simulink library "qrd_matrix_library"  (Simulink 8.7)
settings: Solver=ode45  StartTime=0.0  StopTime=10.0  RelTol=1e-3
values from neighbouring files (symbols this model uses):
  vectorization = 2    [qrd_test.m]
undefined symbols (not defined in the file or in its folder): AdvDSPBChannelOutDisplay, AdvDSPBDMemDisplay, Back_Substitution_instances, column_count, column_count_1, column_count_2, dpoly, dspba_ChannelInVis, dspba_ChannelOutVis, dspba_internal_get_channel_ports, evalAionMaskParam, latency, primtype, QRD_vectorization, recipsqrt, row, row_count, row_count_1, row_count_2, UseDontCare, value, x
libraries: DSPBAPrim x683, DSPBAControl x37, qrd_matrix_library x33, DSPBAVectorUtil x6, DSPBAVectorPrim x3
(part 1 of 8)
settings Model: Creator=idf-2016  LastModifiedBy=5g

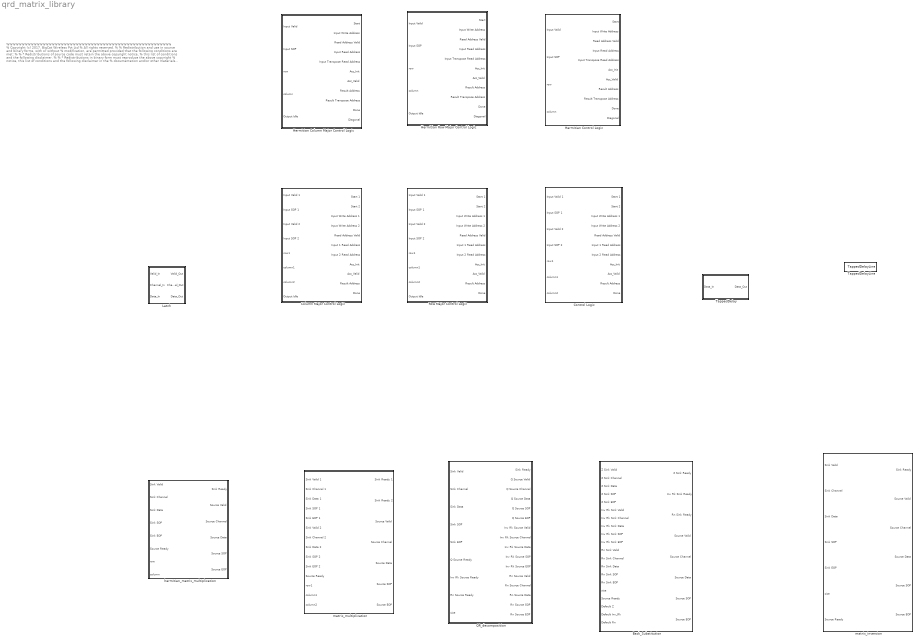
== system qrd_matrix_library ==
  note: %%%%%%%%%%%%%%%%%%%%%%%%%%%%%%%%%%%%%%%%%%%%%%%%%%%%%%%
      |  % Copyright (c) 2017, BigCat Wireless Pvt Ltd
      |  % All rights reserved.
      |  %
      |  % Redistribution and use in source and binary forms, with or without
      |  % modification, are permitted provided that the following conditions are met:
      |  %
      |  %     * Redistributions of source code must retain the above copyright notice,
      |  %       this list of conditions and the following disclaimer.
      |  %
      |  %     * Redistributions in binary form must reproduce the above copyright
      |  %       notice, this list of conditions and the following disclaimer in the
      |  %       documentation and/or other materials provided with the distribution.
      |  %
      |  %     * Neither the name of the copyright holder nor the names of its contributors
      |  %       may be used to endorse or promote products derived from this software
      |  %       without specific prior written permission.
      |  %
      |  %
      |  %
      |  % THIS SOFTWARE IS PROVIDED BY THE COPYRIGHT HOLDERS AND CONTRIBUTORS "AS IS"
      |  % AND ANY EXPRESS OR IMPLIED WARRANTIES, INCLUDING, BUT NOT LIMITED TO, THE
      |  % IMPLIED WARRANTIES OF MERCHANTABILITY AND FITNESS FOR A PARTICULAR PURPOSE ARE
      |  % DISCLAIMED. IN NO EVENT SHALL THE COPYRIGHT HOLDER OR CONTRIBUTORS BE LIABLE
      |  % FOR ANY DIRECT, INDIRECT, INCIDENTAL, SPECIAL, EXEMPLARY, OR CONSEQUENTIAL
      |  % DAMAGES (INCLUDING, BUT NOT LIMITED TO, PROCUREMENT OF SUBSTITUTE GOODS OR
      |  % SERVICES; LOSS OF USE, DATA, OR PROFITS; OR BUSINESS INTERRUPTION) HOWEVER
      |  % CAUSED AND ON ANY THEORY OF LIABILITY, WHETHER IN CONTRACT, STRICT LIABILITY,
      |  % OR TORT (INCLUDING NEGLIGENCE OR OTHERWISE) ARISING IN ANY WAY OUT OF THE USE
      |  % OF THIS SOFTWARE, EVEN IF ADVISED OF THE POSSIBILITY OF SUCH DAMAGE.
      |  %
      |   %%%%%%%%%%%%%%%%%%%%%%%%%%%%%%%%%%%%%%%%%%%%%%%%%%%%%%%%%%
  Back_Substitution : Subsystem  mask{size=16, instances=4}
      mask prompts: size "Number of Unknowns"; instances "Number of Instances"
  Column Major Control Logic : Subsystem
  Control Logic : Subsystem  BlockChoice=Row Major Control Logic
      settings: TemplateBlock=self  MemberBlocks=Column Major Control Logic,Row Major Control Logic
  Hermitian Column Major Control Logic : Subsystem
  Hermitian Control Logic : Subsystem  BlockChoice=Hermitian Column Major Control Logic
      settings: TemplateBlock=self  MemberBlocks=Hermitian Column Major Control Logic,Hermitian Row Major Control Logic
  Hermitian Row Major Control Logic : Subsystem
  Latch : Subsystem
  QR_decomposition : Subsystem  mask{size=16, vectorization=2}
      mask prompts: size "Size of Matrix"
      mask init:
      | %Output_Word_Length = get_param(gcb,'Output_Word_Length');
      | [f,e]=log2(size);
      | if(f ~= 0.5)
      |     if(vectorization~=1)
      |         vectorization = 1;
      |         set_param(gcb,'vectorization','1');
      |         uiwait(msgbox({'Vectorization not allowed for matrix size non powers of 2';'Setting vectorization to 1'},'Vectorization error','error'));
      |     end
      | end
      | 
      | if(vectorization~=1)
      |     [f,e]=log2(vectorization);
      |     if(f ~= 0.5)
      |         vectorization = 1;
      |         set_param(gcb,'vectorization','1');
      |         uiwait(msgbox({'Non power of 2 Vectorization value not allowed';'Setting vectorization to 1'},'Vectorization error','error'));
      |     elseif(vectorization > size)
      |         vectorization = column_count;
      |         set_param(gcb,'vectorization',num2str(vectorization));
      |         uiwait(msgbox({'Vectorization should be less than matrix size';'Setting vectorization equal to matrix size'},'Vectorization error','error'));
      |     end
      | end
  Row Major Control Logic : Subsystem
  TappedDelay : Subsystem  mask{numTaps=2}
      mask prompts: numTaps "Number of Taps"
      mask init:
      | block = gcb;
      | 
      | % This block modifies itself
      | set_param(block, 'MaskSelfModifiable', 'on');
      | % delete all current connections
      | delete_line(find_system(block, 'SearchDepth', 1,...
      |             'FollowLinks', 'on', 'LookUnderMasks', 'all',...
      |             'FindAll', 'on', 'Type', 'line'));
      |         
      | % If there are any SamnpleDelays, delete them
      | delay = find_system(block, 'SearchDepth', 1,...
      |             'FollowLinks', 'on', 'LookUnderMasks', 'all',...
      |             'ReferenceBlock', 'DSPBAPrim/SampleDelay');
      | if ~isempty(delay)
      |     delete_block(delay);
      | end
      | 
      | % Delete the Simulink mux (by name)
      | if ~isempty(find_system(block, 'SearchDepth', 1,...
      |             'FollowLinks', 'on', 'LookUnderMasks', 'all',...
      |             'Name', 'Mux'))
      |         delete_block([block '/Mux']);
      | end
      | 
      | % Now have an empty subsystem cleared of any previous parameterization 
      | % add in the new blocks
      | 
      | if (numTaps <= 1)
      |     % No taps
      |     add_line(block, 'Data_In/1', 'Data_Out/1', 'AUTOROUTING','ON');
      | else
      |     % First a zero-latency or single-latency latch
      |     tdspacing = min(100,(2^14)/numTaps);
      |     tdspacing_half = tdspacing/2;
      |     tdlatchheight = min(40,tdspacing);
      |     
      |     for n=1:(numTaps-1)
      |         add_block('DSPBAPrim/SampleDelay', [block '/tap' num2str(n)],'value',int2str(numTaps-n), 'Position', [130, 220 + tdspacing*n, 190, 220 + tdlatchheight + tdspacing*n]);
      |     end
      |     % Then the Simulink Mux
      |     add_block('built-in/Mux', [block '/Mux'], 'Inputs', int2str(numTaps), 'DisplayOption', 'bar');
      |     set_param([block '/Mux'], 'Position', [335, 190, 345, 190 + numTaps * tdspacing]);
      | 
      |     % Position the ports
      |     set_param([block '/Data_In'], 'Position',  [65,  135, 95,  150]);
      |     set_param([block '/Data_Out'],  'Position', [400,(180 + tdspacing_half*numTaps), 430, (195 + tdspacing_half*numTaps )]);
      | 
      | 
      |     % Now to connect - data chain
      |     add_line(block, 'Data_In/1', sprintf('Mux/%d', numTaps), 'AUTOROUTING','ON');
      |     for n=1:(numTaps-1)
      |         add_line(block, 'Data_In/1', sprintf('tap%d/1', n), 'AUTOROUTING','ON');
      |     end
      | 
      |     % Now to connect the mux to the output
      |     add_line(block, 'Mux/1', 'Data_Out/1');
      |  
      |     % Now to connect - chain to mux
      |     for n=1:(numTaps-1)
      |         add_line(block, sprintf('tap%d/1', n), sprintf('Mux/%d', n));
      |     end
      | end
  TappedDelayLine : DSPBAVectorUtil/TappedDelayLine  numTaps=Back_Substitution_instances/QRD_vectorization  zeroOrOne=0  reverse=on
  hermitian_matrix_multiplication : Subsystem  mask{row_count=16, column_count=32, vectorization=2, output_order=Row Major}
      mask prompts: row_count "Number of Rows"; column_count "Number of Columns"; output_order "Output order"
      mask init:
      | %Output_Word_Length = get_param(gcb,'Output_Word_Length');
      | [f,e]=log2(column_count);
      | if(f ~= 0.5)
      |     if(vectorization~=1)
      |         vectorization = 1;
      |         set_param(gcb,'vectorization','1');
      |         uiwait(msgbox({'Vectorization not allowed for column count non powers of 2';'Setting vectorization to 1'},'Vectorization error','error'));
      |     end
      | end
      | 
      | if(vectorization~=1)
      |     [f,e]=log2(vectorization);
      |     if(f ~= 0.5)
      |         vectorization = 1;
      |         set_param(gcb,'vectorization','1');
      |         uiwait(msgbox({'Non power of 2 Vectorization value not allowed';'Setting vectorization to 1'},'Vectorization error','error'));
      |     elseif(vectorization > column_count)
      |         vectorization = column_count;
      |         set_param(gcb,'vectorization',num2str(vectorization));
      |         uiwait(msgbox({'Vectorization should be less than column count';'Setting vectorization equal to column count'},'Vectorization error','error'));
      |     end
      | end
      | 
      | if(output_order==1)
      |     set_param([gcb '/Hermitian Control Logic'],'BlockChoice','Hermitian Row Major Control Logic');
      | elseif(output_order==2)
      |     set_param([gcb '/Hermitian Control Logic'],'BlockChoice','Hermitian Column Major Control Logic');
      | end
      mask TypeOptions output_order: Row Major | Column Major
  matrix_inversion : Subsystem  mask{size=16, QRD_vectorization=2, Back_Substitution_instances=4}
      mask prompts: size "Size of Matrix"; QRD_vectorization "Vectorization"; Back_Substitution_instances "Number of Instances"
      mask DialogControl QRDGroupVar Prompt: QR Decomposition
      mask DialogControl BSGroupVar Prompt: BackSubstitution
  matrix_multiplication : Subsystem  mask{row_count_1=16, column_count_1=16, row_count_2=16, column_count_2=32, vectorization=4, output_order=Row Major}
      mask prompts: row_count_1 "Number of Rows"; column_count_1 "Number of Columns"; row_count_2 "Number of Rows"; column_count_2 "Number of Columns"; output_order "Output order"
      mask init:
      | %Output_Word_Length = get_param(gcb,'Output_Word_Length');
      | 
      | if(column_count_1~=row_count_2)
      |     row_count_2 = column_count_1;
      |     set_param(gcb,'row_count_2',num2str(row_count_2));
      |     uiwait(msgbox({'Matrix 2 row should be equal to Matrix 1 column';'Setting Matrix 2 row equal to Matrix 1 column'},'Dimension error','error'));
      | end
      | 
      | [f,e]=log2(column_count_1);
      | if(f ~= 0.5)
      |     if(vectorization~=1)
      |         vectorization = 1;
      |         set_param(gcb,'vectorization','1');
      |         uiwait(msgbox({'Vectorization not allowed for Matrix 1 column count non powers of 2';'Setting vectorization to 1'},'Vectorization error','error'));
      |     end
      | end
      | 
      | if(vectorization~=1)
      |     [f,e]=log2(vectorization);
      |     if(f ~= 0.5)
      |         vectorization = 1;
      |         set_param(gcb,'vectorization','1');
      |         uiwait(msgbox({'Non power of 2 Vectorization value not allowed';'Setting vectorization to 1'},'Vectorization error','error'));
      |     elseif(vectorization > column_count_1)
      |         vectorization = column_count_1;
      |         set_param(gcb,'vectorization',num2str(vectorization));
      |         uiwait(msgbox({'Vectorization should be less than Matrix 1 column count';'Setting vectorization equal to column count'},'Vectorization error','error'));
      |     end
      | end
      | 
      | if(output_order==1)
      |     set_param([gcb '/Control Logic'],'BlockChoice','Row Major Control Logic');
      | elseif(output_order==2)
      |     set_param([gcb '/Control Logic'],'BlockChoice','Column Major Control Logic');
      | end
      mask TypeOptions output_order: Row Major | Column Major
      mask DialogControl Matrix1GroupVar Prompt: Matrix 1
      mask DialogControl Matrix2GroupVar Prompt: Matrix 2

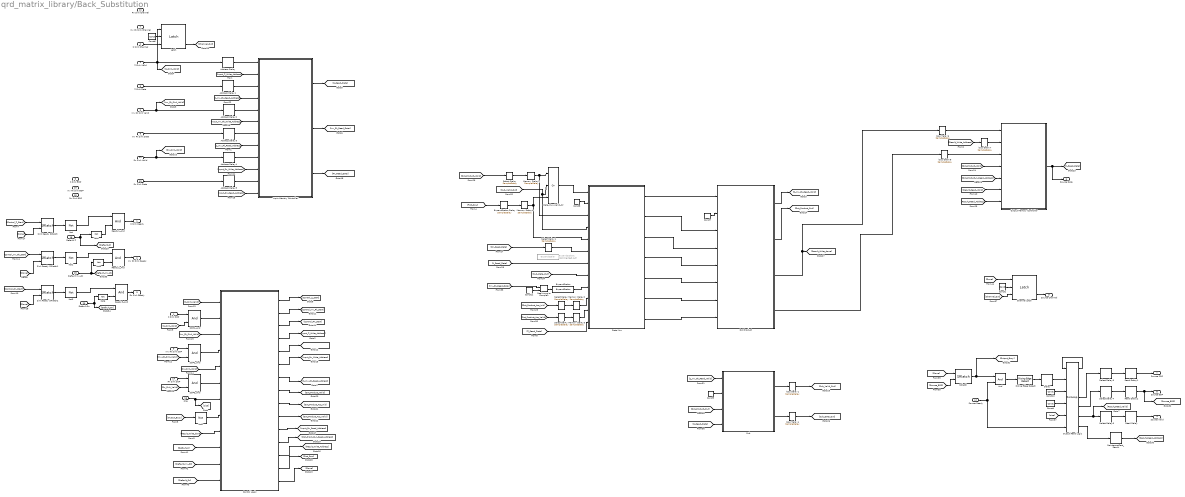
== system qrd_matrix_library/Back_Substitution ==
  Z Sink Valid : Inport
  Z Sink Channel : Inport  Port=2
  Z Sink Data : Inport  Port=3
  Z Sink SOP : Inport  Port=4
  Z Sink EOP : Inport  Port=5
  Inv Rk Sink Valid : Inport  Port=6
  Inv Rk Sink Channel : Inport  Port=7
  Inv Rk Sink Data : Inport  Port=8
  Inv Rk Sink SOP : Inport  Port=9
  Inv Rk Sink EOP : Inport  Port=10
  Rn Sink Valid : Inport  Port=11
  Rn Sink Channel : Inport  Port=12
  Rn Sink Data : Inport  Port=13
  Rn Sink SOP : Inport  Port=14
  Rn Sink EOP : Inport  Port=15
  size : Inport  Port=16
  Source Ready : Inport  Port=17
  Default Z : Inport  Port=18
  Default Inv_Rk : Inport  Port=19
  Default Rn : Inport  Port=20
  Address Delay{,1..5} (6 alike) : DSPBAPrim/SampleDelay  primtype=sampdelay  nInputs=1  nOutputs=1  omode=Inherit via internal rule  otype=sfix(16)  scale=2^-15  rndmethod=Unbiased  factor=1  satmethod=Symmetric  shift_vec=[0 1 2 -1]  value=1  inPortNames=[' '; ' ';]  outPortNames=[' ']  dspbaimage=dspba_prim.jpg  text=dpoly(1, eye(1,value+1), 'z')  style=Optimised  visibilities=8 + 1024 + 2^17 + 2^18  flexible=off  slackgroup=0  augmented=0  version=20090407  advOptions=[]
  And : DSPBAPrim/And  primtype=and  nInputs=2  nOutputs=1  omode=Inherit via internal rule  otype=sfix(16)  scale=2^-15  rndmethod=Unbiased  factor=1  satmethod=Symmetric  shift_vec=[0 1 2 -1]  value=0  inPortNames=[' '; ' '; ' '; ' '; ' '; ' '; ' '; ' '; ' '; ' '; ' '; ' '; ' '; ' '; ' '; ' '; ]  outPortNames=[' ']  dspbaimage=dspba_prim.jpg  text=fprintf('&');  style=Optimised  visibilities=8+2  version=20090407
  Channel Latch : qrd_matrix_library/Latch
  Const{1,6..9} (5 alike) : DSPBAPrim/Const  primtype=const  nInputs=0  nOutputs=1  omode=Specify via dialog  otype=uint(8)  scale=1  rndmethod=Unbiased  factor=1  satmethod=Symmetric  shift_vec=[0 1 2 -1]  value=0  inPortNames=['+'; '+';]  outPortNames=[' ']  dspbaimage=dspba_prim.jpg  text=fprintf('%s', num2str(value));  style=Optimised  visibilities=8 + 1024  floatPrecision=float32_m23  version=20120820
  Const10 : DSPBAPrim/Const  primtype=const  nInputs=0  nOutputs=1  omode=Specify via dialog  otype=uint(nextpow2(size))  scale=1  rndmethod=Unbiased  factor=1  satmethod=Symmetric  shift_vec=[0 1 2 -1]  value=0  inPortNames=['+'; '+';]  outPortNames=[' ']  dspbaimage=dspba_prim.jpg  text=fprintf('%s', num2str(value));  style=Optimised  visibilities=8 + 1024  floatPrecision=float32_m23  version=20120820
  Const11 : DSPBAPrim/Const  primtype=const  nInputs=0  nOutputs=1  omode=single  otype=uint(8)  scale=1  rndmethod=Unbiased  factor=1  satmethod=Symmetric  shift_vec=[0 1 2 -1]  value=0  inPortNames=['+'; '+';]  outPortNames=[' ']  dspbaimage=dspba_prim.jpg  text=fprintf('%s', num2str(value));  style=Optimised  visibilities=8 + 1024  floatPrecision=float32_m23  version=20120820
  Const4 : DSPBAPrim/Const  primtype=const  nInputs=0  nOutputs=1  omode=Inherit via internal rule  otype=uint(nextpow2(row*row))  scale=1  rndmethod=Unbiased  factor=1  satmethod=Symmetric  shift_vec=[0 1 2 -1]  value=1  inPortNames=['+'; '+';]  outPortNames=[' ']  dspbaimage=dspba_prim.jpg  text=fprintf('%s', num2str(value));  style=Optimised  visibilities=8 + 1024  floatPrecision=float32_m23  version=20120820
  Control Logic : Subsystem
  Data Mux : Subsystem
  Data_Mux_Valid_Or : DSPBAPrim/Or  primtype=or  nInputs=3  nOutputs=1  omode=Inherit via internal rule  otype=sfix(16)  scale=2^-15  rndmethod=Unbiased  factor=1  satmethod=Symmetric  shift_vec=[0 1 2 -1]  value=0  inPortNames=[' '; ' '; ' '; ' '; ' '; ' '; ' '; ' '; ' '; ' '; ' '; ' '; ' '; ' '; ' '; ' '; ]  outPortNames=[' ']  dspbaimage=dspba_prim.jpg  text=fprintf('|');  style=Optimised  visibilities=8+2  version=20090407
  Delay : DSPBAPrim/SampleDelay  primtype=sampdelay  nInputs=1  nOutputs=1  omode=Inherit via internal rule  otype=sfix(16)  scale=2^-15  rndmethod=Unbiased  factor=1  satmethod=Symmetric  shift_vec=[0 1 2 -1]  value=1  inPortNames=[' '; ' ';]  outPortNames=[' ']  dspbaimage=dspba_prim.jpg  text=dpoly(1, eye(1,value+1), 'z')  style=Optimised  visibilities=8 + 1024 + 2^17 + 2^18  flexible=off  slackgroup=0  augmented=0  version=20090407  advOptions=[]
  Dot Product : Subsystem
  ExpandScalar : DSPBAVectorUtil/ExpandScalar  vecWidth=instances
  ExpandScalar Delay : DSPBAPrim/SampleDelay  primtype=sampdelay  nInputs=1  nOutputs=1  omode=Inherit via internal rule  otype=sfix(16)  scale=2^-15  rndmethod=Unbiased  factor=1  satmethod=Symmetric  shift_vec=[0 1 2 -1]  value=1  inPortNames=[' '; ' ';]  outPortNames=[' ']  dspbaimage=dspba_prim.jpg  text=dpoly(1, eye(1,value+1), 'z')  style=Optimised  visibilities=8 + 1024 + 2^17 + 2^18  flexible=off  slackgroup=0  augmented=0  version=20090407  advOptions=[]
  ExpandScalar1 : DSPBAVectorUtil/ExpandScalar  Commented=on  vecWidth=instances
  Input Memory Controller : Subsystem
  Latch : qrd_matrix_library/Latch
  Memory Delay{1..4} (4 alike) : DSPBAPrim/SampleDelay  primtype=sampdelay  nInputs=1  nOutputs=1  omode=Inherit via internal rule  otype=sfix(16)  scale=2^-15  rndmethod=Unbiased  factor=1  satmethod=Symmetric  shift_vec=[0 1 2 -1]  value=2  inPortNames=[' '; ' ';]  outPortNames=[' ']  dspbaimage=dspba_prim.jpg  text=dpoly(1, eye(1,value+1), 'z')  style=Optimised  visibilities=8 + 1024 + 2^17 + 2^18  flexible=off  slackgroup=0  augmented=0  version=20090407  advOptions=[]
  Not{,1..6} (7 alike) : DSPBAPrim/Not  primtype=not  nInputs=1  nOutputs=1  omode=Inherit via internal rule  otype=sfix(16)  scale=2^-15  rndmethod=Unbiased  factor=1  satmethod=Symmetric  shift_vec=[0 1 2 -1]  value=0  inPortNames=[' '; ' ';]  outPortNames=[' ']  dspbaimage=dspba_prim.jpg  text=fprintf('~');  style=Optimised  visibilities=8  version=20090407
  Output Memory Controller : Subsystem
  Output Read Logic : DSPBAPrim/ForLoop  looptest=<
  Read Delay : DSPBAPrim/SampleDelay  primtype=sampdelay  nInputs=1  nOutputs=1  omode=Inherit via internal rule  otype=sfix(16)  scale=2^-15  rndmethod=Unbiased  factor=1  satmethod=Symmetric  shift_vec=[0 1 2 -1]  value=2  inPortNames=[' '; ' ';]  outPortNames=[' ']  dspbaimage=dspba_prim.jpg  text=dpoly(1, eye(1,value+1), 'z')  style=Optimised  visibilities=8 + 1024 + 2^17 + 2^18  flexible=off  slackgroup=0  augmented=0  version=20090407  advOptions=[]
  Read Delay1 : DSPBAPrim/SampleDelay  primtype=sampdelay  nInputs=1  nOutputs=1  omode=Inherit via internal rule  otype=sfix(16)  scale=2^-15  rndmethod=Unbiased  factor=1  satmethod=Symmetric  shift_vec=[0 1 2 -1]  value=2  inPortNames=[' '; ' ';]  outPortNames=[' ']  dspbaimage=dspba_prim.jpg  text=dpoly(1, eye(1,value+1), 'z')  style=Optimised  visibilities=8 + 1024 + 2^17 + 2^18  flexible=off  slackgroup=0  augmented=0  version=20090407  advOptions=[]
  Read Delay2 : DSPBAPrim/SampleDelay  primtype=sampdelay  nInputs=1  nOutputs=1  omode=Inherit via internal rule  otype=sfix(16)  scale=2^-15  rndmethod=Unbiased  factor=1  satmethod=Symmetric  shift_vec=[0 1 2 -1]  value=2  inPortNames=[' '; ' ';]  outPortNames=[' ']  dspbaimage=dspba_prim.jpg  text=dpoly(1, eye(1,value+1), 'z')  style=Optimised  visibilities=8 + 1024 + 2^17 + 2^18  flexible=off  slackgroup=0  augmented=0  version=20090407  advOptions=[]
  Ready1_And : DSPBAPrim/And  primtype=and  nInputs=2  nOutputs=1  omode=Inherit via internal rule  otype=sfix(16)  scale=2^-15  rndmethod=Unbiased  factor=1  satmethod=Symmetric  shift_vec=[0 1 2 -1]  value=0  inPortNames=[' '; ' '; ' '; ' '; ' '; ' '; ' '; ' '; ' '; ' '; ' '; ' '; ' '; ' '; ' '; ' '; ]  outPortNames=[' ']  dspbaimage=dspba_prim.jpg  text=fprintf('&');  style=Optimised  visibilities=8+2  version=20090407
  Ready2_And : DSPBAPrim/And  primtype=and  nInputs=2  nOutputs=1  omode=Inherit via internal rule  otype=sfix(16)  scale=2^-15  rndmethod=Unbiased  factor=1  satmethod=Symmetric  shift_vec=[0 1 2 -1]  value=0  inPortNames=[' '; ' '; ' '; ' '; ' '; ' '; ' '; ' '; ' '; ' '; ' '; ' '; ' '; ' '; ' '; ' '; ]  outPortNames=[' ']  dspbaimage=dspba_prim.jpg  text=fprintf('&');  style=Optimised  visibilities=8+2  version=20090407
  Ready3_And : DSPBAPrim/And  primtype=and  nInputs=2  nOutputs=1  omode=Inherit via internal rule  otype=sfix(16)  scale=2^-15  rndmethod=Unbiased  factor=1  satmethod=Symmetric  shift_vec=[0 1 2 -1]  value=0  inPortNames=[' '; ' '; ' '; ' '; ' '; ' '; ' '; ' '; ' '; ' '; ' '; ' '; ' '; ' '; ' '; ' '; ]  outPortNames=[' ']  dspbaimage=dspba_prim.jpg  text=fprintf('&');  style=Optimised  visibilities=8+2  version=20090407
  Real-Imag to Complex : RealImagToComplex
  ReinterpretCast_Result : DSPBAPrim/ReinterpretCast  primtype=reinterpret  nInputs=1  nOutputs=1  omode=Specify via dialog  otype=uint(nextpow2(size))  scale=1  rndmethod=Unbiased  factor=1  satmethod=Symmetric  shift_vec=[0 1 2 -1]  value=0  inPortNames=[' '; ' ';]  outPortNames=[' ']  dspbaimage=dspba_prim.jpg  text=fprintf('Reinterp\nCast', value);  style=Optimised  visibilities=8  floatPrecision=float32_m23  version=20120601
  Rising Edge Detect : qrd_matrix_library/matrix_multiplication/Rising Edge Detect
  SOP1_And : DSPBAPrim/And  primtype=and  nInputs=2  nOutputs=1  omode=Inherit via internal rule  otype=sfix(16)  scale=2^-15  rndmethod=Unbiased  factor=1  satmethod=Symmetric  shift_vec=[0 1 2 -1]  value=0  inPortNames=[' '; ' '; ' '; ' '; ' '; ' '; ' '; ' '; ' '; ' '; ' '; ' '; ' '; ' '; ' '; ' '; ]  outPortNames=[' ']  dspbaimage=dspba_prim.jpg  text=fprintf('&');  style=Optimised  visibilities=8+2  version=20090407
  SOP2_And : DSPBAPrim/And  primtype=and  nInputs=2  nOutputs=1  omode=Inherit via internal rule  otype=sfix(16)  scale=2^-15  rndmethod=Unbiased  factor=1  satmethod=Symmetric  shift_vec=[0 1 2 -1]  value=0  inPortNames=[' '; ' '; ' '; ' '; ' '; ' '; ' '; ' '; ' '; ' '; ' '; ' '; ' '; ' '; ' '; ' '; ]  outPortNames=[' ']  dspbaimage=dspba_prim.jpg  text=fprintf('&');  style=Optimised  visibilities=8+2  version=20090407
  SOP3_And : DSPBAPrim/And  primtype=and  nInputs=2  nOutputs=1  omode=Inherit via internal rule  otype=sfix(16)  scale=2^-15  rndmethod=Unbiased  factor=1  satmethod=Symmetric  shift_vec=[0 1 2 -1]  value=0  inPortNames=[' '; ' '; ' '; ' '; ' '; ' '; ' '; ' '; ' '; ' '; ' '; ' '; ' '; ' '; ' '; ' '; ]  outPortNames=[' ']  dspbaimage=dspba_prim.jpg  text=fprintf('&');  style=Optimised  visibilities=8+2  version=20090407
  SRlatch : DSPBAControl/SRlatch
  Select Delay{,1..6} (7 alike) : DSPBAPrim/SampleDelay  primtype=sampdelay  nInputs=1  nOutputs=1  omode=Inherit via internal rule  otype=sfix(16)  scale=2^-15  rndmethod=Unbiased  factor=1  satmethod=Symmetric  shift_vec=[0 1 2 -1]  value=1  inPortNames=[' '; ' ';]  outPortNames=[' ']  dspbaimage=dspba_prim.jpg  text=dpoly(1, eye(1,value+1), 'z')  style=Optimised  visibilities=8 + 1024 + 2^17 + 2^18  flexible=off  slackgroup=0  augmented=0  version=20090407  advOptions=[]
  Sink Ready SRlatch : DSPBAControl/SRlatch
  Sink Ready SRlatch1 : DSPBAControl/SRlatch
  Sink Ready SRlatch2 : DSPBAControl/SRlatch
  Sub : Subsystem
  loop Delay{1,4,6..8} (5 alike) : DSPBAPrim/SampleDelay  primtype=sampdelay  nInputs=1  nOutputs=1  omode=Inherit via internal rule  otype=sfix(16)  scale=2^-15  rndmethod=Unbiased  factor=1  satmethod=Symmetric  shift_vec=[0 1 2 -1]  value=1  inPortNames=[' '; ' ';]  outPortNames=[' ']  dspbaimage=dspba_prim.jpg  text=dpoly(1, eye(1,value+1), 'z')  style=Optimised  visibilities=8 + 1024 + 2^17 + 2^18  flexible=off  slackgroup=0  augmented=0  version=20090407  advOptions=[]
  Z Sink Ready : Outport
  Inv Rk Sink Ready : Outport  Port=2
  Rn Sink Ready : Outport  Port=3
  Source Valid : Outport  Port=4
  Source Channel : Outport  Port=5
  Source Data : Outport  Port=6
  Source SOP : Outport  Port=7
  Source EOP : Outport  Port=8
  wires:
  Address Delay/1 -> Input Memory Controller/1(Z External Write)
  Z Sink Data/1 -> Address Delay1/1
  Control Logic/4(Z Input Write Address) -> [Input_Z_Write_Address]
  Address Delay1/1 -> Input Memory Controller/3(Z External Write Data)
  [Input_Z_Write_Address] -> Input Memory Controller/2(Z External Write Address)
  Z Sink SOP/1 -> SOP1_And/1
  [Z_Inv_Rk_Read_Address] -> Input Memory Controller/4(Z Read Address)
  [Z_Inv_Rk_Read_Address] -> Input Memory Controller/8(Inv Rk Read Address)
  Z Sink Valid/1 -> Latch/1, Address Delay/1, [Z_Sink_Valid]
  Not/1 -> Ready1_And/1
  [Done] -> Sink Ready SRlatch/2
  Z Sink Channel/1 -> Latch/3
  Const6/1 -> Latch/2
  Latch/3 -> [Channel_Out]
  Sink Ready SRlatch/1 -> Not/1
  [Z_Sink_Valid] -> SOP1_And/2
  SOP1_And/1 -> Control Logic/2(Z Input SOP)
  Control Logic/1(Z Start) -> [Control_Z_Start]
  Not1/1 -> Ready2_And/1
  [Done] -> Sink Ready SRlatch1/2
  Sink Ready SRlatch1/1 -> Not1/1
  [Control_Inv_Rk_Start] -> Sink Ready SRlatch1/1
  Address Delay2/1 -> Input Memory Controller/5(Inv Rk External Write)
  Inv Rk Sink Valid/1 -> [Inv_Rk_Sink_Valid], Address Delay2/1
  Address Delay3/1 -> Input Memory Controller/7(Inv Rk External Write Data)
  Inv Rk Sink Data/1 -> Address Delay3/1
  [Inv_Rk_Sink_Valid] -> SOP2_And/2
  Inv Rk Sink SOP/1 -> SOP2_And/1
  [Z_Sink_Valid] -> Control Logic/1(Z Input Valid)
  [Inv_Rk_Sink_Valid] -> Control Logic/3(Inv Rk Input Valid)
  SOP2_And/1 -> Control Logic/4(Inv Rk Input SOP)
  size/1 -> [size], Control Logic/7(size)
  Control Logic/2(Inv Rk Start) -> [Control_Inv_Rk_Start]
  [Input_Inv_Rk_Write_Address] -> Input Memory Controller/6(Inv Rk External Write Address)
  Control Logic/5(Inv Rk Input Write Address) -> [Input_Inv_Rk_Write_Address]
  [Output_Busy] -> Not2/1
  Not2/1 -> Control Logic/8(Output Idle)
  Rn Sink Valid/1 -> [Rn_Sink_Valid], Address Delay4/1
  Rn Sink Data/1 -> Address Delay5/1
  Address Delay4/1 -> Input Memory Controller/9(Rn External Write)
  Address Delay5/1 -> Input Memory Controller/11(Rn External Write Data)
  Not3/1 -> Ready3_And/1
  [Done] -> Sink Ready SRlatch2/2
  Sink Ready SRlatch2/1 -> Not3/1
  [Control_Rn_Start] -> Sink Ready SRlatch2/1
  [Rn_Sink_Valid] -> SOP3_And/2
  SOP3_And/1 -> Control Logic/6(Rn Input SOP)
  Rn Sink SOP/1 -> SOP3_And/1
  [Rn_Sink_Valid] -> Control Logic/5(Rn Input Valid)
  Control Logic/3(Rn Start) -> [Control_Rn_Start]
  Control Logic/6(Rn Input Write Address) -> [Input_Rn_Write_Address]
  [Input_Rn_Write_Address] -> Input Memory Controller/10(Rn External Write Address)
  Control Logic/7(Z Inv_Rk Read Address) -> [Z_Inv_Rk_Read_Address]
  [Input_Rn_Read_Address] -> Input Memory Controller/12(Rn Read Address)
  Control Logic/13(Result Write Address) -> [Result_Write_Address]
  Input Memory Controller/1(Z Data) -> [Z_Read_Data]
  Input Memory Controller/2(Inv Rk Data) -> [Inv_Rk_Read_Data]
  Control Logic/15(Done) -> [Done]
  Const7/1 -> Dot Product/2(Channel_In)
  Data Mux/4(Acc_Init_Out) -> Dot Product/5(Acc_Init)
  Data Mux/2(Data Out 1) -> Dot Product/3(Data_In1)
  Data Mux/1(Valid Out) -> Dot Product/1(Valid_In)
  Data Mux/3(Data Out 2) -> Dot Product/4(Data_In2)
  Data Mux/5(Acc_Valid_Out) -> Dot Product/6(Acc_Valid)
  Control Logic/11(Rn Read Address) -> [Input_Rn_Read_Address]
  Input Memory Controller/3(Rn Data) -> [Rn_Read_Data]
  Control Logic/12(X Read Address) -> [Dot_Product_X_Read_Address]
  Control Logic/8(Dot Product Valid) -> [Dot_Product_Valid]
  Control Logic/9(Acc_Init) -> [Dot_Product_Acc_Init]
  Control Logic/10(Acc_Valid) -> [Dot_Product_Acc_Valid]
  [Dot_Product_Valid] -> Output Memory Controller/4(Read Valid 1)
  [Result_Read_Valid] -> Output Memory Controller/6(Read Valid 2)
  [Result_Read_Address] -> Output Memory Controller/7(Read Address 2)
  [Dot_Product_X_Read_Address] -> Output Memory Controller/5(Read Address 1)
  Output Memory Controller/1(Read Data) -> Source Data/1, [X_Read_Data]
  Memory Delay1/1 -> Data Mux/3(Dot_Product_valid_in), Data_Mux_Valid_Or/1
  [Sub_Valid_Out] -> Data Mux/4(Divide_valid_in), Data_Mux_Valid_Or/2
  Data_Mux_Valid_Or/1 -> Data Mux/1(Valid In)
  Select Delay/1 -> Memory Delay1/1
  Const8/1 -> Data Mux/2(Channel In)
  Select Delay2/1 -> Memory Delay2/1
  Select Delay3/1 -> Memory Delay3/1
  Memory Delay2/1 -> Data Mux/10(Acc_Init_In)
  Memory Delay3/1 -> Data Mux/11(Acc_Valid_In)
  Dot Product/1(Dot Product Valid_Out) -> [Z_Inv_Rk_Read_Valid]
  Dot Product/2(Dot Product Data_Out) -> [Dot_Product_Out]
  [Sub_Data_Out] -> Data Mux/8(Sub_Data)
  [Inv_Rk_Read_Data] -> Real-Imag to Complex/1
  [Z_Inv_Rk_Read_Valid] -> Sub/1(Valid In)
  Const9/1 -> Sub/2(Channel In)
  [Z_Read_Data] -> Sub/4(Z_Data_In)
  [Dot_Product_Out] -> Sub/3(Acc_Data_In)
  Sub/1(Valid_out) -> loop Delay1/1
  Sub/2(Z_Acc_Data_Out) -> loop Delay4/1
  [Result_Write_done] -> Control Logic/9(Result write done)
  Data Mux/7(Divide_Valid_Out) -> Dot Product/8(Mult_Valid_In)
  Const11/1 -> Real-Imag to Complex/2
  Real-Imag to Complex/1 -> ExpandScalar/1
  ExpandScalar/1 -> Data Mux/9(Inv_Rk_Data)
  [Rn_Read_Data] -> Select Delay1/1
  Dot Product/3(Mult Valid_out) -> loop Delay6/1, [Result_Write_done]
  [Result_Write_Address] -> loop Delay7/1
  Dot Product/4(Mult Data_out) -> loop Delay8/1
  [X_Read_Data] -> Data Mux/7(X_Data)
  Select Delay1/1 -> Data Mux/6(Rn_Data)
  [Dot_Product_Valid] -> Select Delay/1
  [Dot_Product_Acc_Init] -> Select Delay2/1
  [Dot_Product_Acc_Valid] -> Select Delay3/1
  loop Delay6/1 -> Output Memory Controller/1(Write Enable)
  loop Delay7/1 -> Output Memory Controller/2(Write Address)
  loop Delay8/1 -> Output Memory Controller/3(Write Data)
  loop Delay1/1 -> [Sub_Valid_Out]
  loop Delay4/1 -> [Sub_Data_Out]
  Control Logic/14(First Row) -> [First_Row]
  Memory Delay4/1 -> Data Mux/5(First_Column_in), Data_Mux_Valid_Or/3
  ExpandScalar Delay/1 -> Memory Delay4/1
  [First_Row] -> ExpandScalar Delay/1
  [Z_Read_Data] -> Data Mux/12(Z_Data_In)
  Data Mux/6(Dot_Product_valid_out) -> Dot Product/7(Dot_Product_Valid_In)
  Read Delay1/1 -> Source SOP/1
  Read Delay/1 -> Source Valid/1
  Source Ready/1 -> Output Read Logic/6, And/2
  Read Delay2/1 -> Source EOP/1, [Source_EOP]
  Rising Edge Detect/1 -> Delay/1
  SRlatch/1 -> [Output_Busy], And/1
  And/1 -> Rising Edge Detect/1
  Delay/1 -> Output Read Logic/2
  Output Read Logic/6 -> Select Delay6/1, [Result_Read_Valid]
  Output Read Logic/7 -> ReinterpretCast_Result/1
  Output Read Logic/4 -> Select Delay5/1
  Output Read Logic/5 -> Select Delay4/1
  [size] -> Output Read Logic/5
  Const4/1 -> Output Read Logic/4
  Output Read Logic/1 -> Output Read Logic/1
  [Source_EOP] -> SRlatch/2
  ReinterpretCast_Result/1 -> [Result_Read_Address]
  [Done] -> SRlatch/1
  Select Delay5/1 -> Read Delay1/1
  Select Delay4/1 -> Read Delay2/1
  Select Delay6/1 -> Read Delay/1
  Const10/1 -> Output Read Logic/3
  Default Z/1 -> [Default_Z], Not4/1
  Default Inv_Rk/1 -> Not5/1, [Default_Inv_Rk]
  Default Rn/1 -> [Default_Rn], Not6/1
  [Default_Z] -> Control Logic/10(Default Z)
  [Default_Inv_Rk] -> Control Logic/11(Default Inv_Rk)
  [Default_Rn] -> Control Logic/12(Default Rn)
  [Control_Z_Start] -> Sink Ready SRlatch/1
  Ready1_And/1 -> Z Sink Ready/1
  Not4/1 -> Ready1_And/2
  Ready2_And/1 -> Inv Rk Sink Ready/1
  Not5/1 -> Ready2_And/2
  Ready3_And/1 -> Rn Sink Ready/1
  Not6/1 -> Ready3_And/2
  [Channel_Out] -> Channel Latch/3
  Const1/1 -> Channel Latch/2
  [Done] -> Channel Latch/1
  Channel Latch/3 -> Source Channel/1

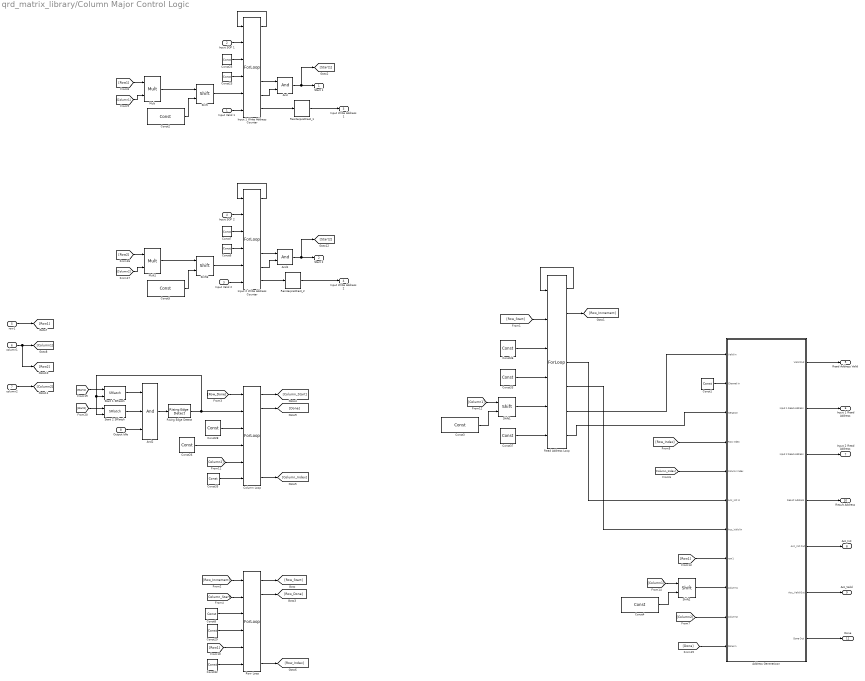
== system qrd_matrix_library/Column Major Control Logic ==
  Input Valid 1 : Inport
  Input SOP 1 : Inport  Port=2
  Input Valid 2 : Inport  Port=3
  Input SOP 2 : Inport  Port=4
  row1 : Inport  Port=5
  column1 : Inport  Port=6
  column2 : Inport  Port=7
  Output Idle : Inport  Port=8
  Address Generatioon : Subsystem
  And : DSPBAPrim/And  primtype=and  nInputs=2  nOutputs=1  omode=Inherit via internal rule  otype=sfix(16)  scale=2^-15  rndmethod=Unbiased  factor=1  satmethod=Symmetric  shift_vec=[0 1 2 -1]  value=0  inPortNames=[' '; ' '; ' '; ' '; ' '; ' '; ' '; ' '; ' '; ' '; ' '; ' '; ' '; ' '; ' '; ' '; ]  outPortNames=[' ']  dspbaimage=dspba_prim.jpg  text=fprintf('&');  style=Optimised  visibilities=8+2  version=20090407
  And1 : DSPBAPrim/And  primtype=and  nInputs=2  nOutputs=1  omode=Inherit via internal rule  otype=sfix(16)  scale=2^-15  rndmethod=Unbiased  factor=1  satmethod=Symmetric  shift_vec=[0 1 2 -1]  value=0  inPortNames=[' '; ' '; ' '; ' '; ' '; ' '; ' '; ' '; ' '; ' '; ' '; ' '; ' '; ' '; ' '; ' '; ]  outPortNames=[' ']  dspbaimage=dspba_prim.jpg  text=fprintf('&');  style=Optimised  visibilities=8+2  version=20090407
  And2 : DSPBAPrim/And  primtype=and  nInputs=3  nOutputs=1  omode=Inherit via internal rule  otype=sfix(16)  scale=2^-15  rndmethod=Unbiased  factor=1  satmethod=Symmetric  shift_vec=[0 1 2 -1]  value=0  inPortNames=[' '; ' '; ' '; ' '; ' '; ' '; ' '; ' '; ' '; ' '; ' '; ' '; ' '; ' '; ' '; ' '; ]  outPortNames=[' ']  dspbaimage=dspba_prim.jpg  text=fprintf('&');  style=Optimised  visibilities=8+2  version=20090407
  Column Loop : DSPBAPrim/ForLoop  looptest=<
  Const1 : DSPBAPrim/Const  primtype=const  nInputs=0  nOutputs=1  omode=Specify via dialog  otype=uint(8)  scale=1  rndmethod=Unbiased  factor=1  satmethod=Symmetric  shift_vec=[0 1 2 -1]  value=0  inPortNames=['+'; '+';]  outPortNames=[' ']  dspbaimage=dspba_prim.jpg  text=fprintf('%s', num2str(value));  style=Optimised  visibilities=8 + 1024  floatPrecision=float32_m23  version=20120820
  Const{2..5} (4 alike) : DSPBAPrim/Const  primtype=const  nInputs=0  nOutputs=1  omode=Inherit via internal rule  otype=uint(8)  scale=1  rndmethod=Unbiased  factor=1  satmethod=Symmetric  shift_vec=[0 1 2 -1]  value=nextpow2(vectorization)  inPortNames=['+'; '+';]  outPortNames=[' ']  dspbaimage=dspba_prim.jpg  text=fprintf('%s', num2str(value));  style=Optimised  visibilities=8 + 1024  floatPrecision=float32_m23  version=20120820
  Const{6,23,26,29,33,35,37} (7 alike) : DSPBAPrim/Const  primtype=const  nInputs=0  nOutputs=1  omode=Inherit via internal rule  otype=uint(8)  scale=1  rndmethod=Unbiased  factor=1  satmethod=Symmetric  shift_vec=[0 1 2 -1]  value=1  inPortNames=['+'; '+';]  outPortNames=[' ']  dspbaimage=dspba_prim.jpg  text=fprintf('%s', num2str(value));  style=Optimised  visibilities=8 + 1024  floatPrecision=float32_m23  version=20120820
  Const{7..8,25,28,36} (5 alike) : DSPBAPrim/Const  primtype=const  nInputs=0  nOutputs=1  omode=Inherit via internal rule  otype=uint(8)  scale=1  rndmethod=Unbiased  factor=1  satmethod=Symmetric  shift_vec=[0 1 2 -1]  value=0  inPortNames=['+'; '+';]  outPortNames=[' ']  dspbaimage=dspba_prim.jpg  text=fprintf('%s', num2str(value));  style=Optimised  visibilities=8 + 1024  floatPrecision=float32_m23  version=20120820
  Const32 : DSPBAPrim/Const  primtype=const  nInputs=0  nOutputs=1  omode=boolean  otype=uint(8)  scale=1  rndmethod=Unbiased  factor=1  satmethod=Symmetric  shift_vec=[0 1 2 -1]  value=1  inPortNames=['+'; '+';]  outPortNames=[' ']  dspbaimage=dspba_prim.jpg  text=fprintf('%s', num2str(value));  style=Optimised  visibilities=8 + 1024  floatPrecision=float32_m23  version=20120820
  Input 1 Write Address Counter : DSPBAPrim/ForLoop  looptest=<
  Input 2 Write Address Counter : DSPBAPrim/ForLoop  looptest=<
  Mult : DSPBAPrim/Mult  primtype=mult  nInputs=2  nOutputs=1  omode=Inherit via internal rule  otype=sfix(16)  scale=2^-15  rndmethod=Unbiased  factor=1  satmethod=Symmetric  shift_vec=[0 1 2 -1]  value=0  inPortNames=[' '; ' ';]  outPortNames=[' ']  dspbaimage=dspba_prim.jpg  text=fprintf('X');  style=Optimised  visibilities=8+2^18+2^19  floatPrecision=float32_m23  floatRounding=correct  advOptions=[]  version=20130115
  Mult1 : DSPBAPrim/Mult  primtype=mult  nInputs=2  nOutputs=1  omode=Inherit via internal rule  otype=sfix(16)  scale=2^-15  rndmethod=Unbiased  factor=1  satmethod=Symmetric  shift_vec=[0 1 2 -1]  value=0  inPortNames=[' '; ' ';]  outPortNames=[' ']  dspbaimage=dspba_prim.jpg  text=fprintf('X');  style=Optimised  visibilities=8+2^18+2^19  floatPrecision=float32_m23  floatRounding=correct  advOptions=[]  version=20130115
  Read Address Loop : DSPBAPrim/ForLoop  looptest=<
  ReinterpretCast_1 : DSPBAPrim/ReinterpretCast  primtype=reinterpret  nInputs=1  nOutputs=1  omode=Specify via dialog  otype=uint(nextpow2((row_count_1*column_count_1)/vectorization))  scale=1  rndmethod=Unbiased  factor=1  satmethod=Symmetric  shift_vec=[0 1 2 -1]  value=0  inPortNames=[' '; ' ';]  outPortNames=[' ']  dspbaimage=dspba_prim.jpg  text=fprintf('Reinterp\nCast', value);  style=Optimised  visibilities=8  floatPrecision=float32_m23  version=20120601
  ReinterpretCast_2 : DSPBAPrim/ReinterpretCast  primtype=reinterpret  nInputs=1  nOutputs=1  omode=Specify via dialog  otype=uint(nextpow2((row_count_2*column_count_2)/vectorization))  scale=1  rndmethod=Unbiased  factor=1  satmethod=Symmetric  shift_vec=[0 1 2 -1]  value=0  inPortNames=[' '; ' ';]  outPortNames=[' ']  dspbaimage=dspba_prim.jpg  text=fprintf('Reinterp\nCast', value);  style=Optimised  visibilities=8  floatPrecision=float32_m23  version=20120601
  Rising Edge Detect : qrd_matrix_library/matrix_multiplication/Rising Edge Detect
  Row Loop : DSPBAPrim/ForLoop  looptest=<
  Shift{,1..3} (4 alike) : DSPBAPrim/Shift  primtype=shift  nInputs=2  nOutputs=1  omode=Inherit via internal rule  otype=sfix(16)  scale=2^-15  rndmethod=Unbiased  factor=1  satmethod=Symmetric  shift_vec=[0 1 2 -1]  value=0  inPortNames=['a'; 'b';]  outPortNames=[' ']  dspbaimage=dspba_prim.jpg  text=fprintf('a >> b');  style=Optimised  visibilities=8  version=20090407
  Start 1 SRlatch : DSPBAControl/SRlatch
  Start 2 SRlatch : DSPBAControl/SRlatch
  Start 1 : Outport
  Start 2 : Outport  Port=2
  Input Write Address 1 : Outport  Port=3
  Input Write Address 2 : Outport  Port=4
  Read Address Valid : Outport  Port=5
  Input 1 Read Address : Outport  Port=6
  Input 2 Read Address : Outport  Port=7
  Acc_Init : Outport  Port=8
  Acc_Valid : Outport  Port=9
  Result Address : Outport  Port=10
  Done : Outport  Port=11
  wires:
  Address Generatioon/7(Done Out) -> Done/1
  [Done] -> Address Generatioon/11(Done In)
  [Row_Start] -> Read Address Loop/2
  Input SOP 1/1 -> Input 1 Write Address Counter/2
  Read Address Loop/2 -> [Row_Increment]
  Input 1 Write Address Counter/6 -> And/2
  Input 1 Write Address Counter/5 -> And/1
  Input 1 Write Address Counter/1 -> Input 1 Write Address Counter/1
  Input Valid 1/1 -> Input 1 Write Address Counter/6
  Shift2/1 -> Address Generatioon/9(column1)
  Const4/1 -> Shift2/2
  [Column1] -> Shift2/1
  [Row1] -> Address Generatioon/8(row1)
  Const3/1 -> Shift1/2
  [Column1] -> Shift1/1
  Const2/1 -> Shift/2
  Mult/1 -> Shift/1
  [Column1] -> Mult/2
  [Row1] -> Mult/1
  column1/1 -> [Row2], [Column1]
  row1/1 -> [Row1]
  Const1/1 -> Address Generatioon/2(Channel In)
  Address Generatioon/5(Acc_Init Out) -> Acc_Init/1
  Address Generatioon/6(Acc_Valid Out) -> Acc_Valid/1
  Read Address Loop/6 -> Address Generatioon/1(Valid In)
  Address Generatioon/4(Result Address) -> Result Address/1
  Address Generatioon/2(Input 1 Read Address) -> Input 1 Read Address/1
  Address Generatioon/3(Input 2 Read Address) -> Input 2 Read Address/1
  [Column_Index] -> Address Generatioon/5(Column Index)
  [Row_Index] -> Address Generatioon/4(Row Index)
  Read Address Loop/7 -> Address Generatioon/3(Iteration)
  Column Loop/2 -> [Done]
  Read Address Loop/5 -> Address Generatioon/7(Acc_Valid In)
  Read Address Loop/4 -> Address Generatioon/6(Acc_Init In)
  Address Generatioon/1(Valid Out) -> Read Address Valid/1
  Row Loop/7 -> [Row_Index]
  Const37/1 -> Read Address Loop/6
  Column Loop/1 -> [Column_Start]
  [Column_Start] -> Row Loop/2
  [Row_Done] -> Column Loop/1
  Row Loop/2 -> [Row_Done]
  [Row_Increment] -> Row Loop/1
  Row Loop/1 -> [Row_Start]
  Const35/1 -> Column Loop/6
  Const32/1 -> Row Loop/6
  Shift1/1 -> Read Address Loop/5
  Const33/1 -> Read Address Loop/4
  Const36/1 -> Read Address Loop/3
  Read Address Loop/1 -> Read Address Loop/1
  Column Loop/7 -> [Column_Index]
  Const29/1 -> Row Loop/4
  [Column2] -> Column Loop/5
  Const28/1 -> Column Loop/3
  Const26/1 -> Column Loop/4
  [Row1] -> Row Loop/5
  Input 1 Write Address Counter/7 -> ReinterpretCast_1/1
  Const25/1 -> Input 1 Write Address Counter/3
  Const23/1 -> Input 1 Write Address Counter/4
  Shift/1 -> Input 1 Write Address Counter/5
  column2/1 -> [Column2]
  Input SOP 2/1 -> Input 2 Write Address Counter/2
  Input 2 Write Address Counter/6 -> And1/2
  Input 2 Write Address Counter/5 -> And1/1
  Input 2 Write Address Counter/1 -> Input 2 Write Address Counter/1
  Input Valid 2/1 -> Input 2 Write Address Counter/6
  Const5/1 -> Shift3/2
  Mult1/1 -> Shift3/1
  [Column2] -> Mult1/2
  [Row2] -> Mult1/1
  Input 2 Write Address Counter/7 -> ReinterpretCast_2/1
  Const7/1 -> Input 2 Write Address Counter/3
  Const6/1 -> Input 2 Write Address Counter/4
  Shift3/1 -> Input 2 Write Address Counter/5
  And/1 -> [Start1], Start 1/1
  And1/1 -> [Start2], Start 2/1
  Const8/1 -> Row Loop/3
  [Column2] -> Address Generatioon/10(column2)
  ReinterpretCast_1/1 -> Input Write Address 1/1
  ReinterpretCast_2/1 -> Input Write Address 2/1
  Rising Edge Detect/1 -> Column Loop/2, Start 1 SRlatch/2, Start 2 SRlatch/2
  [Start1] -> Start 1 SRlatch/1
  [Start2] -> Start 2 SRlatch/1
  And2/1 -> Rising Edge Detect/1
  Output Idle/1 -> And2/3
  Start 1 SRlatch/1 -> And2/1
  Start 2 SRlatch/1 -> And2/2

== system qrd_matrix_library/Control Logic ==
  Input Valid 1 : Inport
  Input SOP 1 : Inport  Port=2
  Input Valid 2 : Inport  Port=3
  Input SOP 2 : Inport  Port=4
  row1 : Inport  Port=5
  column1 : Inport  Port=6
  column2 : Inport  Port=7
  Row Major Control Logic : qrd_matrix_library/Row Major Control Logic
  Start 1 : Outport
  Start 2 : Outport  Port=2
  Input Write Address 1 : Outport  Port=3
  Input Write Address 2 : Outport  Port=4
  Read Address Valid : Outport  Port=5
  Input 1 Read Address : Outport  Port=6
  Input 2 Read Address : Outport  Port=7
  Acc_Init : Outport  Port=8
  Acc_Valid : Outport  Port=9
  Result Address : Outport  Port=10
  Done : Outport  Port=11
  wires:
  Input Valid 1/1 -> Row Major Control Logic/1
  Input SOP 1/1 -> Row Major Control Logic/2
  Input Valid 2/1 -> Row Major Control Logic/3
  Input SOP 2/1 -> Row Major Control Logic/4
  row1/1 -> Row Major Control Logic/5
  column1/1 -> Row Major Control Logic/6
  column2/1 -> Row Major Control Logic/7
  Row Major Control Logic/1 -> Start 1/1
  Row Major Control Logic/2 -> Start 2/1
  Row Major Control Logic/3 -> Input Write Address 1/1
  Row Major Control Logic/4 -> Input Write Address 2/1
  Row Major Control Logic/5 -> Read Address Valid/1
  Row Major Control Logic/6 -> Input 1 Read Address/1
  Row Major Control Logic/7 -> Input 2 Read Address/1
  Row Major Control Logic/8 -> Acc_Init/1
  Row Major Control Logic/9 -> Acc_Valid/1
  Row Major Control Logic/10 -> Result Address/1
  Row Major Control Logic/11 -> Done/1
